simulink model "QuadrotorSimulink_w_memory_z_desired_inzemam"  (R2020a)
settings: Solver=FixedStepAuto  StartTime=0.0  StopTime=options.T_train  FixedStep=options.dt  RelTol=1e-6
undefined symbols (not defined in the file or in its folder): options, Quad
libraries: neural x125, simulink x3
(part 4 of 7)

== system QuadrotorSimulink_w_memory_z_desired_inzemam/NN/Layer 2/Delays 1 ==
  "p{2}" : Inport  PortDimensions=50
      mask Display: e = 0.06;c1 = [120 230 180]/255;c2 = ([120 230 180]+0)/(256+128);c3 = ([120 230 180]+128)/(256+128);patch([0 1 1 0],[0 0 1 1],c1);patch([0 1 1 1-e 1-e 0+e],[0 0 1 1-e 0+e 0+e],c2);patch([0 0 1 1-e 0+e 0+e],[0 1 1 1-e 1-e 0+e],c3);plot([0 1 1 0 0],[0 0 1 1 0]);
  mux : Mux  Inputs=1
      mask Display: e = 0.06;c1 = [120 150 230]/255;c2 = ([120 150 230]+0)/383;c3 = ([120 150 230]+128)/383;patch([0 1 1 0],[0 0 1 1],c1);patch([0 1 1 1-e 1-e 0+e],[0 0 1 1-e 0+e 0+e],c2);patch([0 0 1 1-e 0+e 0+e],[0 1 1 1-e 1-e 0+e],c3);plot([0 1 1 0 0],[0 0 1 1 0]);disp('Mux')
  "pd{2,1}" : Outport
      mask Display: e = 0.06;c1 = [120 230 180]/255;c2 = ([120 230 180]+0)/(256+128);c3 = ([120 230 180]+128)/(256+128);patch([0 1 1 0],[0 0 1 1],c1);patch([0 1 1 1-e 1-e 0+e],[0 0 1 1-e 0+e 0+e],c2);patch([0 0 1 1-e 0+e 0+e],[0 1 1 1-e 1-e 0+e],c3);plot([0 1 1 0 0],[0 0 1 1 0]);
  wires:
  "p{2}"/1 -> mux/1
  mux/1 -> "pd{2,1}"/1

== system QuadrotorSimulink_w_memory_z_desired_inzemam/NN/Layer 2/LW{2,1} ==
  "ad{2,1}" : Inport  PortDimensions=50
      mask Display: e = 0.06;c1 = [120 230 180]/255;c2 = ([120 230 180]+0)/(256+128);c3 = ([120 230 180]+128)/(256+128);patch([0 1 1 0],[0 0 1 1],c1);patch([0 1 1 1-e 1-e 0+e],[0 0 1 1-e 0+e 0+e],c2);patch([0 0 1 1-e 0+e 0+e],[0 1 1 1-e 1-e 0+e],c3);plot([0 1 1 0 0],[0 0 1 1 0]);
  "IW{2,1}(1,:)'" : Constant  Value=[-0.2180991707686248670672313210161519236862659454345703125;0.6034435892571303750031574963941238820552825927734375;0.1448570765852514596883082731437752954661846160888671875;-0.0919104607025376385553983027421054430305957794189453125;-0.254834546036511289113235534387058578431606292724609375;-0.0289448614546063721919555433714776881970465183258056640625;-0.005912785822548833995770944937930835294537246227264404296875;0.0514572024798022609193282050910056568682193756103515625;0.1617687360125932560794836945206043310463428497314453125;-0.06296832164801713371815594655345194041728973388671875;0.354822168982281638260900535897235386073589324951171875;-0.207949222529742072662628515899996273219585418701171875;0.043548527376515384912369910352936130948364734649658203125;0.09218733860702645055429371723221265710890293121337890625;-0.298471195843326764229885839085909537971019744873046875;-0.2126003988632956254178907329333014786243438720703125;-0.31752734092446843749968365955282934010028839111328125;0.25682876579573932218636400648392736911773681640625;0.0491195778741810029632830492118955589830875396728515625;-0.045571709983612519734297308104942203499376773834228515625;-0.01743945921805532817128181477528414689004421234130859375;0.1281628956757363824170425914417137391865253448486328125;-0.040103129045937657704001821912243030965328216552734375;0.55129480172784040004074768148711882531642913818359375;0.1826795755725003633784808698692359030246734619140625;-0.1273691719002043309938443371720495633780956268310546875;0.1344931238994332145519905452601960860192775726318359375;-0.041885711089975748155911361436665174551308155059814453125;-0.0222800743292805546180712639170451438985764980316162109375;0.07901018825114773658224720520593109540641307830810546875;-0.032702424582651663798049668230305542238056659698486328125;-0.054991984881678883378963718087106826715171337127685546875;0.305063413395850135945153169814147986471652984619140625;0.1516498793852104898238764008056023158133029937744140625;0.2678918157044141157285821464029140770435333251953125;0.0007986938890895416316706434400884973001666367053985595703125;0.1503256643881707710352912954476778395473957061767578125;-0.337238309906441546814903631457127630710601806640625;-0.11443690423163367653192068473799736239016056060791015625;-0.09679156389455290110390706104226410388946533203125;0.00438002043409591555744864166399565874598920345306396484375;-0.06751244271055979739859509436428197659552097320556640625;0.3126354595164213545643860925338231027126312255859375;-0.21316673877165082107154603363596834242343902587890625;0.54568611006834999432868471558322198688983917236328125;0.08763704288126128449931684372131712734699249267578125;0.1266642393785563369679181278115720488131046295166015625;-0.324847899901827996682612820222857408225536346435546875;-0.11338354816450306461472763430720078758895397186279296875;-0.422647560179592207685317362120258621871471405029296875]
      mask Display: e = 0.06;c1 = [120 150 230]/255;c2 = ([120 150 230]+0)/383;c3 = ([120 150 230]+128)/383;patch([0 1 1 0],[0 0 1 1],c1);patch([0 1 1 1-e 1-e 0+e],[0 0 1 1-e 0+e 0+e],c2);patch([0 0 1 1-e 0+e 0+e],[0 1 1 1-e 1-e 0+e],c3);plot([0 1 1 0 0],[0 0 1 1 0]);disp('weights');
  "IW{2,1}(2,:)'" : Constant  Value=[-0.034857291084589049623421175283510820008814334869384765625;-0.237953352169493370649178132225642912089824676513671875;0.1347969287081599298883105575441732071340084075927734375;-0.0077593975109727063299569493892704485915601253509521484375;-0.165131951309862079479984231511480174958705902099609375;0.1899049032826858052214191729945014230906963348388671875;0.1867380133697902622191833188480813987553119659423828125;-0.2016620844103868270824619912673369981348514556884765625;0.0987485734057493846904662859742529690265655517578125;0.0890766748615987591364273612271063029766082763671875;-0.06716907710615760418448871860164217650890350341796875;-0.09145894292547292192541164013164234347641468048095703125;-0.1364666284510190619183589433305314742028713226318359375;0.1742046475753933065799827772934804670512676239013671875;-0.1419274761422510688912979048836859874427318572998046875;-0.0866681828405911069967970661309664137661457061767578125;-0.25630239567824919522109894387540407478809356689453125;0.1380198493045983465510317955704522319138050079345703125;-0.0657758778760896556381254640655242837965488433837890625;-0.07045999201023389613141034715226851403713226318359375;0.0084656185126084915193445112890913151204586029052734375;0.051803630831342005469419831342747784219682216644287109375;0.058383979483588366310442552276072092354297637939453125;-0.031102123658624129809435743254653061740100383758544921875;-0.1824852173521370468645130813456489704549312591552734375;0.0456917528932702932120690775263938121497631072998046875;0.1048677899500579380198672652113600634038448333740234375;0.25191201682447583731772056125919334590435028076171875;0.057334549423298068748788836046514916233718395233154296875;0.002794894326943439359645093844619623268954455852508544921875;-0.134879940658568620026613871232257224619388580322265625;0.03974094186703654163483889760755118913948535919189453125;0.07157935777618397443777809030507341958582401275634765625;0.1408449648934377573805676320262136869132518768310546875;0.119343955202142637528339719210634939372539520263671875;-0.139056748900801607771171575222979299724102020263671875;0.00681364542000185806347456463072376209311187267303466796875;0.048277001421795952273985363945030258037149906158447265625;0.0735884580161776102880111238846438936889171600341796875;0.27584223147199715686639365230803377926349639892578125;0.033477095691278456468520374755826196633279323577880859375;0.0543426655504478384184352535157813690602779388427734375;0.12796587390000191408745422450010664761066436767578125;0.2475284804682862382918528965092264115810394287109375;0.27862163873681300430007468094117939472198486328125;0.1430696322988034008272251185189816169440746307373046875;0.08351432740353124939414186655994853936135768890380859375;0.1330049884976134411118664502282626926898956298828125;-0.170324952189159273263641125595313496887683868408203125;-0.284299864706883453902008795921574346721172332763671875]
      mask Display: e = 0.06;c1 = [120 150 230]/255;c2 = ([120 150 230]+0)/383;c3 = ([120 150 230]+128)/383;patch([0 1 1 0],[0 0 1 1],c1);patch([0 1 1 1-e 1-e 0+e],[0 0 1 1-e 0+e 0+e],c2);patch([0 0 1 1-e 0+e 0+e],[0 1 1 1-e 1-e 0+e],c3);plot([0 1 1 0 0],[0 0 1 1 0]);disp('weights');
  "IW{2,1}(3,:)'" : Constant  Value=[-0.306648076262070856667918405946693383157253265380859375;-0.06582487196319279643130784052118542604148387908935546875;-0.000560457772041487588439434563980512393754906952381134033203125;-0.061433170365345957097957807491184212267398834228515625;0.262408266737736373119815880272653885185718536376953125;-0.09442273888695561223638463843599311076104640960693359375;0.01126600066513742948171028501747059635818004608154296875;-0.016249715370910265688220164292943081818521022796630859375;-0.00786370440059175161706672696482200990431010723114013671875;-0.14717886332263796500541275236173532903194427490234375;-0.01232654273458870519686314537466387264430522918701171875;0.09826358990756924038922903719139867462217807769775390625;-0.09221047666301988854353766100757638923823833465576171875;0.0507075248925279165046475782219204120337963104248046875;-0.114846696354321486932548168624634854495525360107421875;-0.086048022126157974742710621285368688404560089111328125;-0.15167328632555687750738115937565453350543975830078125;0.1112094652968962649186579483284731395542621612548828125;-0.048599804431721523034770626736644771881401538848876953125;0.31434620503736432350905261046136729419231414794921875;-0.034652148184443905265528229620031197555363178253173828125;0.20138503656609552106004912275238893926143646240234375;0.11789565941850564667614520431015989743173122406005859375;0.11531905614543071225686077241334714926779270172119140625;0.12839463314187626874485204098164103925228118896484375;-0.169509938501154200363174595622695051133632659912109375;-0.20431736668476940810279529614490456879138946533203125;0.173469684925514899820342407110729254782199859619140625;-0.081513152966969870671931630567996762692928314208984375;0.07474184147996977556349662563661695457994937896728515625;-0.0722018577210766510088291170177399180829524993896484375;-0.055076765786222114940073879552073776721954345703125;-0.280192490924994597190078593484940938651561737060546875;-0.10618754479733048812217788281486718915402889251708984375;-0.129856706441404068375078395547461695969104766845703125;-0.126591869856962746521134022259502671658992767333984375;-0.304866568414732863612215396642568521201610565185546875;0.357509328536810000453982638646266423165798187255859375;0.264267368666721846892642133752815425395965576171875;-0.2173655624022493848546133676791214384138584136962890625;0.108796541731620788340251237968914210796356201171875;-0.0041566238798640374463300162233281298540532588958740234375;0.2919134177086395443012634132173843681812286376953125;0.1955731229219974665056724916212260723114013671875;0.09380207375614797726814941825068672187626361846923828125;0.0035030693734600924262034826739409254514612257480621337890625;-0.2006454766260882538464471736006089486181735992431640625;0.2477733616744739464365920866839587688446044921875;0.07077756001817959996547102718977839685976505279541015625;-0.1884786659099315364596094468652154318988323211669921875]
      mask Display: e = 0.06;c1 = [120 150 230]/255;c2 = ([120 150 230]+0)/383;c3 = ([120 150 230]+128)/383;patch([0 1 1 0],[0 0 1 1],c1);patch([0 1 1 1-e 1-e 0+e],[0 0 1 1-e 0+e 0+e],c2);patch([0 0 1 1-e 0+e 0+e],[0 1 1 1-e 1-e 0+e],c3);plot([0 1 1 0 0],[0 0 1 1 0]);disp('weights');
  "IW{2,1}(4,:)'" : Constant  Value=[0.01030904375679848362923340943098082789219915866851806640625;-0.33294167500815785576406824475270695984363555908203125;0.2437784724727011520517550025033415295183658599853515625;-0.3158324578265183646408331696875393390655517578125;0.173847042722556910376852101762779057025909423828125;0.318800915191999656439492127901758067309856414794921875;-0.101386120761538023327119617533753626048564910888671875;0.121828945837945123997769769630394876003265380859375;-0.110748113821379112753362505827681161463260650634765625;-0.253305697867314438820329769441741518676280975341796875;-0.341917963226958387945586537171038798987865447998046875;-0.306898886523132852222062183500383980572223663330078125;0.29606081489642266380002411096938885748386383056640625;-0.379436652721030276413927140310988761484622955322265625;-0.01349057438434595780629710048970082425512373447418212890625;-0.07992996381570298403129726239058072678744792938232421875;0.1968973272707283672655620421210187487304210662841796875;0.3089168042076411158092241748818196356296539306640625;0.102544505519770012824665172956883907318115234375;0.217989723561201331758496735346852801740169525146484375;0.11676719845795578700542449723798199556767940521240234375;0.04706051499239481683556363122988841496407985687255859375;0.020006669998177899205682450656240689568221569061279296875;-0.11673929114264959550073541549863875843584537506103515625;0.0480408331255211262789117654392612166702747344970703125;-0.36197990495132270627465231882524676620960235595703125;-0.335821312078860956251702418740023858845233917236328125;-0.0251495087624837472539685023775746230967342853546142578125;0.1770719300736879053825845176106668077409267425537109375;-0.06807299265384143815982298519884352572262287139892578125;0.1398857730715728775461315080974600277841091156005859375;-0.2353875182183125802648504532044171355664730072021484375;-0.193261743316708589635055659528006799519062042236328125;0.043023437828039912123045951375388540327548980712890625;-0.07437840217642786855289926961631863377988338470458984375;0.11341241877907189128382725584742729552090167999267578125;-0.046550247179447001855123744462616741657257080078125;-0.001751611751338556614843167125172840314917266368865966796875;-0.16347020669850864660332945277332328259944915771484375;0.0226077261360675095536176826271912432275712490081787109375;0.1947521562692689223172948231876944191753864288330078125;-0.202593836776758795537034529843367636203765869140625;0.0164860307840504587140184611371296341530978679656982421875;0.035614664236682046227766562651595450006425380706787109375;0.0565438091225107519743886541618849150836467742919921875;-0.22497919149810663430599788625841028988361358642578125;-0.386506869067798131123225857663783244788646697998046875;0.253627325841210116141866137695615179836750030517578125;-0.164598985902752514842717346255085431039333343505859375;-0.282768349972814136972232290645479224622249603271484375]
      mask Display: e = 0.06;c1 = [120 150 230]/255;c2 = ([120 150 230]+0)/383;c3 = ([120 150 230]+128)/383;patch([0 1 1 0],[0 0 1 1],c1);patch([0 1 1 1-e 1-e 0+e],[0 0 1 1-e 0+e 0+e],c2);patch([0 0 1 1-e 0+e 0+e],[0 1 1 1-e 1-e 0+e],c3);plot([0 1 1 0 0],[0 0 1 1 0]);disp('weights');
  Mux : Mux
      mask Display: e = 0.06;c1 = [120 150 230]/255;c2 = ([120 150 230]+0)/383;c3 = ([120 150 230]+128)/383;patch([0 1 1 0],[0 0 1 1],c1);patch([0 1 1 1-e 1-e 0+e],[0 0 1 1-e 0+e 0+e],c2);patch([0 0 1 1-e 0+e 0+e],[0 1 1 1-e 1-e 0+e],c3);plot([0 1 1 0 0],[0 0 1 1 0]);disp('Mux');
  dotprod{1..4} (4 alike) : neural/Weight Functions/dotprod
  "lz{2,1}" : Outport
      mask Display: e = 0.06;c1 = [120 230 180]/255;c2 = ([120 230 180]+0)/(256+128);c3 = ([120 230 180]+128)/(256+128);patch([0 1 1 0],[0 0 1 1],c1);patch([0 1 1 1-e 1-e 0+e],[0 0 1 1-e 0+e 0+e],c2);patch([0 0 1 1-e 0+e 0+e],[0 1 1 1-e 1-e 0+e],c3);plot([0 1 1 0 0],[0 0 1 1 0]);
  wires:
  "IW{2,1}(1,:)'"/1 -> dotprod1/1
  "ad{2,1}"/1 -> dotprod1/2, dotprod2/2, dotprod3/2, dotprod4/2
  dotprod1/1 -> Mux/1
  "IW{2,1}(2,:)'"/1 -> dotprod2/1
  dotprod2/1 -> Mux/2
  "IW{2,1}(3,:)'"/1 -> dotprod3/1
  dotprod3/1 -> Mux/3
  "IW{2,1}(4,:)'"/1 -> dotprod4/1
  dotprod4/1 -> Mux/4
  Mux/1 -> "lz{2,1}"/1

== system QuadrotorSimulink_w_memory_z_desired_inzemam/NN_online/Layer 1/Delays 1 ==
  "p{1}" : Inport  PortDimensions=20
      mask Display: e = 0.06;c1 = [120 230 180]/255;c2 = ([120 230 180]+0)/(256+128);c3 = ([120 230 180]+128)/(256+128);patch([0 1 1 0],[0 0 1 1],c1);patch([0 1 1 1-e 1-e 0+e],[0 0 1 1-e 0+e 0+e],c2);patch([0 0 1 1-e 0+e 0+e],[0 1 1 1-e 1-e 0+e],c3);plot([0 1 1 0 0],[0 0 1 1 0]);
  mux : Mux  Inputs=1
      mask Display: e = 0.06;c1 = [120 150 230]/255;c2 = ([120 150 230]+0)/383;c3 = ([120 150 230]+128)/383;patch([0 1 1 0],[0 0 1 1],c1);patch([0 1 1 1-e 1-e 0+e],[0 0 1 1-e 0+e 0+e],c2);patch([0 0 1 1-e 0+e 0+e],[0 1 1 1-e 1-e 0+e],c3);plot([0 1 1 0 0],[0 0 1 1 0]);disp('Mux')
  "pd{1,1}" : Outport
      mask Display: e = 0.06;c1 = [120 230 180]/255;c2 = ([120 230 180]+0)/(256+128);c3 = ([120 230 180]+128)/(256+128);patch([0 1 1 0],[0 0 1 1],c1);patch([0 1 1 1-e 1-e 0+e],[0 0 1 1-e 0+e 0+e],c2);patch([0 0 1 1-e 0+e 0+e],[0 1 1 1-e 1-e 0+e],c3);plot([0 1 1 0 0],[0 0 1 1 0]);
  wires:
  "p{1}"/1 -> mux/1
  mux/1 -> "pd{1,1}"/1
